simulink model "test_com_SensorFusion_SF_E10_fuerE9Daten"  (R2019b)
settings: Solver=FixedStepDiscrete  StartTime=0  StopTime=85  FixedStep=0.001  RelTol=1e-3
undefined symbols (not defined in the file or in its folder): BxTM, ByTM, CxTM, CyTM, g, gamma_stat_front, gamma_stat_rear, gearbox_ratio, l_F, l_R, m_sprung, m_unsprung_quarter, mag_calib_front_center, mag_calib_front_compmatrix, mag_calib_rear_center, mag_calib_rear_compmatrix, param, switch_VelYcalculation_pSF, testStart_VelX_pSF, testVelY_pSF, tire_r_dyn, track_angle_front, track_width_front, track_width_rear, v2o_x, wheel_kinematics_breakpoints, wheel_kinematics_FL_data, wheel_kinematics_FR_data, wheelbase, x9DFrontX, x9DFrontY, x9DRearX, x9DRearY
libraries: SignalProcessingSensorFusionLib x30, simulink x3
(part 3 of 7)

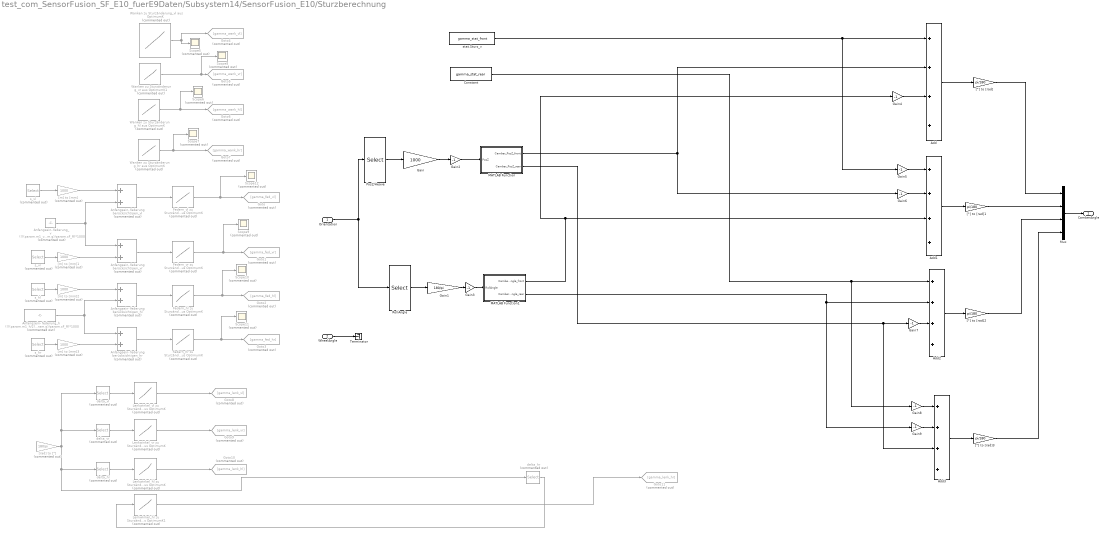
== system test_com_SensorFusion_SF_E10_fuerE9Daten/Subsystem14/SensorFusion_E10/Sturzberechnung ==
  Orientation : Inport
  WheelAngle : Inport  Port=2
  Add{,1..3} (4 alike) : Sum  Inputs=++++
  Anfangsein- federung berücksichtigen_hl : Sum  Commented=on
  Anfangsein- federung berücksichtigen_hr : Sum  Commented=on
  Anfangsein- federung berücksichtigen_vl : Sum  Commented=on
  Anfangsein- federung berücksichtigen_vr : Sum  Commented=on
  Anfangsein- federung_h : Constant  Commented=on  Value=((((param.m1_h/2)+param.m2)*param.g)/param.cF_R)*1000
  Anfangsein- federung_v : Constant  Commented=on  Value=((((param.m1_v/2)+param.m2)*param.g)/param.cF_R)*1000
  Constant : Constant  Value=gamma_stat_rear
  Federn_hl zu Sturzänderung_hl aus OptimumK : Lookup_n-D  Commented=on  NumberOfTableDimensions=1  BreakpointsForDimension1=|  Table=|  InternalRulePriority=Speed  RndMeth=Simplest  InputSameDT=on
      BreakpointsForDimension1=|
      | [-40
      | -37.25
      | -34.5
      | -31.75
      | -29
      | -26.25
      | -23.5
      | -20.75
      | -18
      | -15.25
      | -12.5
      | -9.75
      | -7
      | -4.25
      | -1.5
      | 1.25
      | 4
      | 6.75
      | 9.5
      | 12.25
      | 15]
      Table=|
      | [-1.883
      | -1.737
      | -1.594
      | -1.453
      | -1.315
      | -1.179
      | -1.045
      | -0.914
      | -0.786
      | -0.659
      | -0.535
      | -0.413
      | -0.294
      | -0.177
      | -0.062
      | 0.051
      | 0.161
      | 0.27
      | 0.375
      | 0.479
      | 0.581]
  Federn_hr zu Sturzänderung_hr aus OptimumK : Lookup_n-D  Commented=on  NumberOfTableDimensions=1  BreakpointsForDimension1=|  Table=|  InternalRulePriority=Speed  RndMeth=Simplest  InputSameDT=on
      BreakpointsForDimension1=|
      | [-40
      | -37.25
      | -34.5
      | -31.75
      | -29
      | -26.25
      | -23.5
      | -20.75
      | -18
      | -15.25
      | -12.5
      | -9.75
      | -7
      | -4.25
      | -1.5
      | 1.25
      | 4
      | 6.75
      | 9.5
      | 12.25
      | 15]
      Table=|
      | [-1.883
      | -1.737
      | -1.594
      | -1.453
      | -1.315
      | -1.179
      | -1.045
      | -0.914
      | -0.786
      | -0.659
      | -0.535
      | -0.413
      | -0.294
      | -0.177
      | -0.062
      | 0.051
      | 0.161
      | 0.27
      | 0.375
      | 0.479
      | 0.581]
  Federn_vl zu Sturzänderung_vl aus OptimumK : Lookup_n-D  Commented=on  NumberOfTableDimensions=1  BreakpointsForDimension1=|  Table=|  InternalRulePriority=Speed  RndMeth=Simplest  InputSameDT=on
      BreakpointsForDimension1=|
      | [-40
      | -37.25
      | -34.5
      | -31.75
      | -29
      | -26.25
      | -23.5
      | -20.75
      | -18
      | -15.25
      | -12.5
      | -9.75
      | -7
      | -4.25
      | -1.5
      | 1.25
      | 4
      | 6.75
      | 9.5
      | 12.25
      | 15]
      Table=|
      | [-1.478
      | -1.362
      | -1.249
      | -1.138
      | -1.028
      | -0.921
      | -0.816
      | -0.713
      | -0.612
      | -0.513
      | -0.416
      | -0.321
      | -0.228
      | -0.137
      | -0.048
      | 0.039
      | 0.125
      | 0.208
      | 0.29
      | 0.369
      | 0.447]
  Federn_vr zu Sturzänderung_vr aus OptimumK : Lookup_n-D  Commented=on  NumberOfTableDimensions=1  BreakpointsForDimension1=|  Table=|  InternalRulePriority=Speed  RndMeth=Simplest  InputSameDT=on
      BreakpointsForDimension1=|
      | [-40
      | -37.25
      | -34.5
      | -31.75
      | -29
      | -26.25
      | -23.5
      | -20.75
      | -18
      | -15.25
      | -12.5
      | -9.75
      | -7
      | -4.25
      | -1.5
      | 1.25
      | 4
      | 6.75
      | 9.5
      | 12.25
      | 15]
      Table=|
      | [-1.478
      | -1.362
      | -1.249
      | -1.138
      | -1.028
      | -0.921
      | -0.816
      | -0.713
      | -0.612
      | -0.513
      | -0.416
      | -0.321
      | -0.228
      | -0.137
      | -0.048
      | 0.039
      | 0.125
      | 0.208
      | 0.29
      | 0.369
      | 0.447]
  Gain : Gain  Gain=1000  OutDataTypeStr=single
  Gain1 : Gain  Gain=180/pi
  Gain{2..9} (8 alike) : Gain  Gain=-1  OutDataTypeStr=single
  Goto : Goto  Commented=on  GotoTag=gamma_fed_vl
  Goto1 : Goto  Commented=on  GotoTag=gamma_fed_vr
  Goto10 : Goto  Commented=on  GotoTag=gamma_lenk_hl
  Goto11 : Goto  Commented=on  GotoTag=gamma_lenk_hr
  Goto2 : Goto  Commented=on  GotoTag=gamma_fed_hl
  Goto3 : Goto  Commented=on  GotoTag=gamma_fed_hr
  Goto4 : Goto  Commented=on  GotoTag=gamma_wank_vl
  Goto5 : Goto  Commented=on  GotoTag=gamma_wank_vr
  Goto6 : Goto  Commented=on  GotoTag=gamma_wank_hl
  Goto7 : Goto  Commented=on  GotoTag=gamma_wank_hr
  Goto8 : Goto  Commented=on  GotoTag=gamma_lenk_vl
  Goto9 : Goto  Commented=on  GotoTag=gamma_lenk_vr
  Lenkwinkel_hl zu Sturzänderung_hl aus OptimumK : Lookup_n-D  Commented=on  NumberOfTableDimensions=1  BreakpointsForDimension1=[-3 0 3]  Table=[-0.1 0 0.1]  InternalRulePriority=Speed  RndMeth=Simplest  InputSameDT=on
  Lenkwinkel_hl zu Sturzänderung_hl aus OptimumK1 : Lookup_n-D  Commented=on  NumberOfTableDimensions=1  BreakpointsForDimension1=[-3 0 3]  Table=[0.1 0 -0.1]  InternalRulePriority=Speed  RndMeth=Simplest  InputSameDT=on
  Lenkwinkel_vl zu Sturzänderung_vl aus OptimumK : Lookup_n-D  Commented=on  NumberOfTableDimensions=1  BreakpointsForDimension1=|  Table=|  InternalRulePriority=Speed  RndMeth=Simplest  InputSameDT=on
      BreakpointsForDimension1=|
      | [-31.315
      | -27.82
      | -24.456
      | -21.198
      | -18.024
      | -14.919
      | -11.868
      | -8.861
      | -5.886
      | -2.935
      | 0
      | 2.928
      | 5.856
      | 8.792
      | 11.744
      | 14.718
      | 17.724
      | 20.769
      | 23.864
      | 27.02
      | 30.249]
      Table=|
      | [-0.307
      | -0.4
      | -0.46
      | -0.49
      | -0.492
      | -0.468
      | -0.42
      | -0.349
      | -0.254
      | -0.138
      | 0
      | 0.16
      | 0.342
      | 0.546
      | 0.772
      | 1.022
      | 1.295
      | 1.594
      | 1.919
      | 2.271
      | 2.654]
  Lenkwinkel_vr zu Sturzänderung_vr aus OptimumK : Lookup_n-D  Commented=on  NumberOfTableDimensions=1  BreakpointsForDimension1=|  Table=|  InternalRulePriority=Speed  RndMeth=Simplest  InputSameDT=on
      BreakpointsForDimension1=|
      | [-30.249
      | -27.02
      | -23.864
      | -20.769
      | -17.724
      | -14.718
      | -11.744
      | -8.792
      | -5.856
      | -2.928
      | 0
      | 2.935
      | 5.886
      | 8.861
      | 11.868
      | 14.919
      | 18.024
      | 21.198
      | 24.457
      | 27.82
      | 31.315]
      Table=|
      | [2.654
      | 2.271
      | 1.919
      | 1.594
      | 1.295
      | 1.022
      | 0.772
      | 0.546
      | 0.342
      | 0.16
      | 0
      | -0.138
      | -0.254
      | -0.349
      | -0.42
      | -0.468
      | -0.492
      | -0.49
      | -0.46
      | -0.4
      | -0.307]
  MATLAB Function : MATLAB Function  TreatAsAtomicUnit=on
  MATLAB Function1 : MATLAB Function  TreatAsAtomicUnit=on
  Mux : Mux
  PosZ/Heave : Selector  InputPortWidth=6  IndexOptions=Index vector (dialog)  Indices=1  OutputSizes=1
  RollAngle : Selector  InputPortWidth=6  IndexOptions=Index vector (dialog)  Indices=3  OutputSizes=1
  Scope{5..12} (8 alike) : Scope  Commented=on
  Terminator : Terminator
  Wanken zu Sturzänderung_hl aus OptimumK : Lookup_n-D  Commented=on  NumberOfTableDimensions=1  BreakpointsForDimension1=|  Table=|  InternalRulePriority=Speed  RndMeth=Simplest  InputSameDT=on
      BreakpointsForDimension1=|
      | [-5
      | -4.5
      | -4
      | -3.5
      | -3
      | -2.5
      | -2
      | -1.5
      | -1
      | -0.5
      | 0
      | 0.5
      | 1
      | 1.5
      | 2
      | 2.5
      | 3
      | 3.5
      | 4
      | 4.5
      | 5]
      Table=|
      | [2.509
      | 2.297
      | 2.076
      | 1.847
      | 1.608
      | 1.361
      | 1.106
      | 0.842
      | 0.569
      | 0.289
      | 0
      | -0.297
      | -0.602
      | -0.915
      | -1.235
      | -1.564
      | -1.901
      | -2.245
      | -2.598
      | -2.958
      | -3.327]
  Wanken zu Sturzänderung_hr aus OptimumK : Lookup_n-D  Commented=on  NumberOfTableDimensions=1  BreakpointsForDimension1=|  Table=|  InternalRulePriority=Speed  RndMeth=Simplest  InputSameDT=on
      BreakpointsForDimension1=|
      | [-5
      | -4.5
      | -4
      | -3.5
      | -3
      | -2.5
      | -2
      | -1.5
      | -1
      | -0.5
      | 0
      | 0.5
      | 1
      | 1.5
      | 2
      | 2.5
      | 3
      | 3.5
      | 4
      | 4.5
      | 5]
      Table=|
      | [-3.327
      | -2.958
      | -2.598
      | -2.245
      | -1.901
      | -1.564
      | -1.235
      | -0.915
      | -0.602
      | -0.297
      | 0
      | 0.289
      | 0.569
      | 0.842
      | 1.106
      | 1.361
      | 1.608
      | 1.847
      | 2.076
      | 2.297
      | 2.509]
  Wanken zu Sturzänderung_vl aus OptimumK : Lookup_n-D  Commented=on  NumberOfTableDimensions=1  BreakpointsForDimension1=|  Table=|  InternalRulePriority=Speed  RndMeth=Simplest  InputSameDT=on
      BreakpointsForDimension1=|
      | [-25.00
      | -22.50
      | -20.00
      | -17.50
      | -15.00
      | -12.50
      | -10.00
      | -7.50
      | -5.00
      | -2.50
      | 0.00
      | 2.50
      | 5.00
      | 7.50
      | 10.00
      | 12.50
      | 15.00
      | 17.50
      | 20.00
      | 22.50
      | 25 ]
      Table=|
      | [-0.83
      | -0.74
      | -0.65
      | -0.56
      | -0.47
      | -0.39
      | -0.30
      | -0.23
      | -0.15
      | -0.07
      | 0.00
      | 0.07
      | 0.14
      | 0.20
      | 0.27
      | 0.33
      | 0.39
      | 0.44
      | 0.50
      | 0.55
      | 0.60]
  Wanken zu Sturzänderung_vr aus OptimumK1 : Lookup_n-D  Commented=on  NumberOfTableDimensions=1  BreakpointsForDimension1=|  Table=|  InternalRulePriority=Speed  RndMeth=Simplest  InputSameDT=on
      BreakpointsForDimension1=|
      | [-5
      | -4.5
      | -4
      | -3.5
      | -3
      | -2.5
      | -2
      | -1.5
      | -1
      | -0.5
      | 0
      | 0.5
      | 1
      | 1.5
      | 2
      | 2.5
      | 3
      | 3.5
      | 4
      | 4.5
      | 5]
      Table=|
      | [-3.719
      | -3.319
      | -2.925
      | -2.537
      | -2.155
      | -1.78
      | -1.411
      | -1.048
      | -0.692
      | -0.343
      | 0
      | 0.336
      | 0.666
      | 0.988
      | 1.304
      | 1.613
      | 1.915
      | 2.209
      | 2.497
      | 2.777
      | 3.05]
  [m] to [mm]{,1..3} (4 alike) : Gain  Commented=on  Gain=1000
  "[rad] to [°]" : Gain  Commented=on  Gain=180/pi
  "[°] to [rad]" : Gain  Gain=pi/180
  "[°] to [rad]1" : Gain  Gain=pi/180  OutDataTypeStr=single
  "[°] to [rad]2" : Gain  Gain=pi/180  OutDataTypeStr=single
  "[°] to [rad]3" : Gain  Gain=pi/180  OutDataTypeStr=single
  delta_hl : Selector  Commented=on  InputPortWidth=4  IndexOptions=Index vector (dialog)  Indices=3  OutputSizes=1
  delta_hr : Selector  Commented=on  InputPortWidth=4  IndexOptions=Index vector (dialog)  Indices=4  OutputSizes=1
  delta_vl : Selector  Commented=on  InputPortWidth=4  IndexOptions=Index vector (dialog)  Indices=1  OutputSizes=1
  delta_vr : Selector  Commented=on  InputPortWidth=4  IndexOptions=Index vector (dialog)  Indices=2  OutputSizes=1
  s_hl : Selector  Commented=on  InputPortWidth=14  IndexOptions=Index vector (dialog)  Indices=9  OutputSizes=1
  s_hr : Selector  Commented=on  InputPortWidth=14  IndexOptions=Index vector (dialog)  Indices=10  OutputSizes=1
  s_vl : Selector  Commented=on  InputPortWidth=14  IndexOptions=Index vector (dialog)  Indices=7  OutputSizes=1
  s_vr : Selector  Commented=on  InputPortWidth=14  IndexOptions=Index vector (dialog)  Indices=8  OutputSizes=1
  stat.Sturz_v : Constant  Value=gamma_stat_front
  CamberAngle : Outport  VectorParamsAs1DForOutWhenUnconnected=off
  wires:
  delta_hr/1 -> Lenkwinkel_hl zu Sturzänderung_hl aus OptimumK1/1
  delta_hl/1 -> Lenkwinkel_hl zu Sturzänderung_hl aus OptimumK/1
  delta_vr/1 -> Lenkwinkel_vr zu Sturzänderung_vr aus OptimumK/1
  delta_vl/1 -> Lenkwinkel_vl zu Sturzänderung_vl aus OptimumK/1
  "[rad] to [°]"/1 -> delta_hl/1, delta_hr/1, delta_vl/1, delta_vr/1
  ? -> Wanken zu Sturzänderung_vl aus OptimumK/1, Wanken zu Sturzänderung_vr aus OptimumK1/1, Wanken zu Sturzänderung_hr aus OptimumK/1, Wanken zu Sturzänderung_hl aus OptimumK/1
  "[°] to [rad]"/1 -> Mux/1
  "[°] to [rad]1"/1 -> Mux/2
  "[°] to [rad]2"/1 -> Mux/3
  "[°] to [rad]3"/1 -> Mux/4
  s_vl/1 -> "[m] to [mm]"/1
  s_vr/1 -> "[m] to [mm]1"/1
  s_hl/1 -> "[m] to [mm]2"/1
  s_hr/1 -> "[m] to [mm]3"/1
  "[m] to [mm]"/1 -> Anfangsein- federung berücksichtigen_vl/1
  Anfangsein- federung_v/1 -> Anfangsein- federung berücksichtigen_vl/2, Anfangsein- federung berücksichtigen_vr/1
  "[m] to [mm]1"/1 -> Anfangsein- federung berücksichtigen_vr/2
  "[m] to [mm]2"/1 -> Anfangsein- federung berücksichtigen_hl/1
  Anfangsein- federung_h/1 -> Anfangsein- federung berücksichtigen_hl/2, Anfangsein- federung berücksichtigen_hr/1
  "[m] to [mm]3"/1 -> Anfangsein- federung berücksichtigen_hr/2
  Anfangsein- federung berücksichtigen_vr/1 -> Federn_vr zu Sturzänderung_vr aus OptimumK/1
  Anfangsein- federung berücksichtigen_vl/1 -> Federn_vl zu Sturzänderung_vl aus OptimumK/1
  Anfangsein- federung berücksichtigen_hl/1 -> Federn_hl zu Sturzänderung_hl aus OptimumK/1
  Anfangsein- federung berücksichtigen_hr/1 -> Federn_hr zu Sturzänderung_hr aus OptimumK/1
  Add/1 -> "[°] to [rad]"/1
  Add1/1 -> "[°] to [rad]1"/1
  Add2/1 -> "[°] to [rad]2"/1
  Add3/1 -> "[°] to [rad]3"/1
  Federn_vl zu Sturzänderung_vl aus OptimumK/1 -> Scope12/1, Goto/1
  Federn_vr zu Sturzänderung_vr aus OptimumK/1 -> Scope9/1, Goto1/1
  Federn_hl zu Sturzänderung_hl aus OptimumK/1 -> Scope10/1, Goto2/1
  Federn_hr zu Sturzänderung_hr aus OptimumK/1 -> Scope11/1, Goto3/1
  Wanken zu Sturzänderung_vl aus OptimumK/1 -> Goto4/1, Scope5/1
  Wanken zu Sturzänderung_hr aus OptimumK/1 -> Scope7/1, Goto7/1
  Wanken zu Sturzänderung_hl aus OptimumK/1 -> Scope6/1, Goto6/1
  Wanken zu Sturzänderung_vr aus OptimumK1/1 -> Scope8/1, Goto5/1
  Lenkwinkel_vl zu Sturzänderung_vl aus OptimumK/1 -> Goto8/1
  Lenkwinkel_hl zu Sturzänderung_hl aus OptimumK1/1 -> Goto11/1
  Lenkwinkel_hl zu Sturzänderung_hl aus OptimumK/1 -> Goto10/1
  Lenkwinkel_vr zu Sturzänderung_vr aus OptimumK/1 -> Goto9/1
  ? -> Add3/4
  MATLAB Function/2(Camber_PosZ_rear) -> Add3/3, Gain7/1
  MATLAB Function1/2(Camber_RollAngle_rear) -> Gain9/1, Add2/2
  Orientation/1 -> RollAngle/1, PosZ/Heave/1
  Gain/1 -> Gain2/1
  PosZ/Heave/1 -> Gain/1
  RollAngle/1 -> Gain1/1
  Gain1/1 -> Gain3/1
  MATLAB Function1/1(Camber_RollAngle_front) -> Gain4/1, Add1/3
  Mux/1 -> CamberAngle/1
  WheelAngle/1 -> Terminator/1
  Gain2/1 -> MATLAB Function/1(PosZ)
  MATLAB Function/1(Camber_PosZ_front) -> Add/2, Gain6/1
  stat.Sturz_v/1 -> Add/1, Gain5/1
  Constant/1 -> Add2/1, Gain8/1
  Gain3/1 -> MATLAB Function1/1(RollAngle)
  Gain4/1 -> Add/3
  Gain5/1 -> Add1/1
  Gain6/1 -> Add1/2
  Gain7/1 -> Add2/3
  Gain8/1 -> Add3/1
  Gain9/1 -> Add3/2

== system test_com_SensorFusion_SF_E10_fuerE9Daten/Subsystem14/SensorFusion_E10/simpleTireLoadEstimation ==
  note: Fz_FL
      | Fz_FR
      | Fz_RL
      | Fz_RR
  VehicleState : Inport
  Bus Selector : BusSelector  OutputSignals=AccX,AccY
  MATLAB Function : MATLAB Function  TreatAsAtomicUnit=on
  MATLAB Function4 : MATLAB Function  TreatAsAtomicUnit=on
  Mux2 : Mux
  Scope : Scope  NumInputPorts=2
  TireLoad : Outport  VectorParamsAs1DForOutWhenUnconnected=off
  wires:
  Bus Selector/2 -> MATLAB Function/2(a_y)  "<AccY>"
  VehicleState/1 -> Bus Selector/1
  Bus Selector/1 -> Scope/1, MATLAB Function4/1(AccX)  "<AccX>"
  Mux2/1 -> TireLoad/1
  MATLAB Function/1(F_z_vl) -> Mux2/1
  MATLAB Function/2(F_z_vr) -> Mux2/2
  MATLAB Function/3(F_z_hl) -> Mux2/3
  MATLAB Function/4(F_z_hr) -> Mux2/4
  MATLAB Function4/1(AccX_out) -> Scope/2, MATLAB Function/1(a_x)

== system test_com_SensorFusion_SF_E10_fuerE9Daten/Subsystem14/SensorFusion_E8_adjusted/SensorFusion ==
  note: DriverInput gelöscht -> bei Bedarf ChWi fragen
  9D front : Inport  SampleTime=0.002
  9D rear : Inport  Port=2  SampleTime=0.002
  v2o velocity : Inport  Port=3
  wheel speeds : Inport  Port=4
  rocker angle : Inport  Port=5
  wheel Torque : Inport  Port=6
  wheel Angle : Inport  Port=7
  Constant : Constant
  Terminator{1..4} (4 alike) : Terminator
  kalman : MATLAB Function  TreatAsAtomicUnit=on  SystemSampleTime=0.002
  VehicleState : Outport  OutDataTypeStr=Bus: control_VehicleState  VectorParamsAs1DForOutWhenUnconnected=off
  wires:
  9D rear/1 -> kalman/2(x9DRear)
  kalman/4(Covariance) -> Terminator3/1
  kalman/1(VehicleState) -> VehicleState/1
  kalman/3(Heading) -> Terminator2/1
  kalman/2(bias) -> Terminator1/1
  kalman/5(z_out) -> Terminator4/1
  9D front/1 -> kalman/1(x9DFront)
  rocker angle/1 -> kalman/5(rockerAngles)  "rockerAngle"
  Constant/1 -> kalman/8(driverInputs)
  v2o velocity/1 -> kalman/3(v2o)
  wheel speeds/1 -> kalman/4(WheelSpeeds)
  wheel Torque/1 -> kalman/6(wheelTorques)
  wheel Angle/1 -> kalman/7(wheelAngles)

== system test_com_SensorFusion_SF_E10_fuerE9Daten/Subsystem14/SensorFusion_E8_adjusted/simple_TireLoadEstimation ==
  note: Fz_FL
      | Fz_FR
      | Fz_RL
      | Fz_RR
  VehicleState : Inport  SampleTime=0.002
  Bus Selector : BusSelector  OutputSignals=AccX,AccY
  MATLAB Function : MATLAB Function  TreatAsAtomicUnit=on
  Mux2 : Mux
  TireLoad : Outport  VectorParamsAs1DForOutWhenUnconnected=off
  wires:
  Bus Selector/2 -> MATLAB Function/2(a_y)  "<AccY>"
  VehicleState/1 -> Bus Selector/1
  Bus Selector/1 -> MATLAB Function/1(a_x)  "<AccX>"
  Mux2/1 -> TireLoad/1
  MATLAB Function/1(F_z_vl) -> Mux2/1
  MATLAB Function/2(F_z_vr) -> Mux2/2
  MATLAB Function/3(F_z_hl) -> Mux2/3
  MATLAB Function/4(F_z_hr) -> Mux2/4

== system test_com_SensorFusion_SF_E10_fuerE9Daten/Subsystem14/SensorFusion_E10/DriverDemand_Generation_LaunchControl/Brake Map ==
  note: Bitte mit den Kennlinien unterhalb der 45 Grad Ursprungsgeraden bleiben, Einfluss auf die PowerLimitation sonst nicht auszuschließen
  note: Verschiedene Standard-Pedalmappings (ohne Geschwindigkeits- und Bremskraftfaktoreinfluss) für unterschiedliche Fahrer
  BrakeTorque : Inport
  Driver : Inport  Port=2
  AlDe : Lookup_n-D  NumberOfTableDimensions=1  BreakpointsForDimension1=[0:0.1:1]  Table=[0:0.1:1]  InternalRulePriority=Speed  RndMeth=Simplest  InputSameDT=on
  FeSch : Lookup_n-D  NumberOfTableDimensions=1  BreakpointsForDimension1=[0:0.1:1]  Table=[0:0.1:1]  InternalRulePriority=Speed  RndMeth=Simplest  InputSameDT=on
  Multiport Switch : MultiPortSwitch  DataPortOrder=Zero-based contiguous  zeroidx=on
  SiRi : Lookup_n-D  NumberOfTableDimensions=1  BreakpointsForDimension1=[0:0.1:1]  Table=[0:0.1:1]  InternalRulePriority=Speed  RndMeth=Simplest  InputSameDT=on
  DriverBrakeTorque : Outport  VectorParamsAs1DForOutWhenUnconnected=off
  wires:
  Multiport Switch/1 -> DriverBrakeTorque/1  "DriverBrakeTorque"
  BrakeTorque/1 -> AlDe/1, SiRi/1, FeSch/1
  FeSch/1 -> Multiport Switch/3
  AlDe/1 -> Multiport Switch/2
  SiRi/1 -> Multiport Switch/4
  Driver/1 -> Multiport Switch/1

== system test_com_SensorFusion_SF_E10_fuerE9Daten/Subsystem14/SensorFusion_E10/DriverDemand_Generation_LaunchControl/Subsystem ==
  Drive Request : Inport
  DrivingMode : Inport  Port=2
  DriverDemand_z : Inport  Port=3
  "Aktiviere AccelPedalLogic nur in AccelModus " : simulink/Logic and Bit Operations/Compare To Constant  relop===  const=3  OutDataTypeStr=boolean
  EntryBedingung für AccelPedalLogic : simulink/Logic and Bit Operations/Compare To Constant  relop===  const=1  OutDataTypeStr=boolean
  LeaveBedingung für AccelPedalLogic : simulink/Logic and Bit Operations/Compare To Constant  relop=>=  const=0.5  OutDataTypeStr=boolean
  Logical Operator : Logic  Inputs=3  AllPortsSameDT=off  OutDataTypeStr=boolean
  AccelPedalEnable : Outport  VectorParamsAs1DForOutWhenUnconnected=off
  wires:
  EntryBedingung für AccelPedalLogic/1 -> Logical Operator/3
  LeaveBedingung für AccelPedalLogic/1 -> Logical Operator/1
  Logical Operator/1 -> AccelPedalEnable/1  "AccelPedalEnable"
  DrivingMode/1 -> "Aktiviere AccelPedalLogic nur in AccelModus "/1
  "Aktiviere AccelPedalLogic nur in AccelModus "/1 -> Logical Operator/2
  DriverDemand_z/1 -> EntryBedingung für AccelPedalLogic/1
  Drive Request/1 -> LeaveBedingung für AccelPedalLogic/1

== system test_com_SensorFusion_SF_E10_fuerE9Daten/Subsystem14/SensorFusion_E10/DriverDemand_Generation_LaunchControl/Totbereich Bremspedal ==
  note: Totbereich Pedale
  Pedal_BrakeRecu_Value : Inport
  Kompensation auf ursprünglichen Wertebereich : Gain  Gain=1/0.95
  Totzone Bremspedal : DeadZone  LowerValue=0  UpperValue=0.05  SaturateOnIntegerOverflow=on
  maximaler Wert durch Totzone : Saturate  UpperLimit=0.95  LowerLimit=0
  BrakeTorque : Outport  VectorParamsAs1DForOutWhenUnconnected=off
  wires:
  maximaler Wert durch Totzone/1 -> Kompensation auf ursprünglichen Wertebereich/1
  Kompensation auf ursprünglichen Wertebereich/1 -> BrakeTorque/1  "BrakeTorque"
  Totzone Bremspedal/1 -> maximaler Wert durch Totzone/1
  Pedal_BrakeRecu_Value/1 -> Totzone Bremspedal/1  "BrakeReq"

== system test_com_SensorFusion_SF_E10_fuerE9Daten/Subsystem14/SensorFusion_E10/DriverDemand_Generation_LaunchControl/Totbereich Gaspedal ==
  Pedal_Accel_Value : Inport
  Gain : Gain
  Kompensation auf ursprünglichen Wertebereich : Gain  Gain=1/0.98
  To Drive Torque : Gain
  Totzone Gaspedal : DeadZone  LowerValue=0  UpperValue=0.02  SaturateOnIntegerOverflow=on
  maximaler Wert durch Totzone : Saturate  UpperLimit=0.98  LowerLimit=0
  Drive Request : Outport  VectorParamsAs1DForOutWhenUnconnected=off
  wires:
  Totzone Gaspedal/1 -> maximaler Wert durch Totzone/1
  Gain/1 -> Totzone Gaspedal/1  "TorqueReq"
  maximaler Wert durch Totzone/1 -> Kompensation auf ursprünglichen Wertebereich/1
  To Drive Torque/1 -> Drive Request/1  "Drive Request"
  Pedal_Accel_Value/1 -> Gain/1
  Kompensation auf ursprünglichen Wertebereich/1 -> To Drive Torque/1
